simulink library "cdsDacKill"  (Simulink 7.5)
settings: Solver=ode45  StartTime=0.0  StopTime=10.0  RelTol=1e-3
settings Model: Creator=rolf.bork  LastModifiedBy=rolf.bork

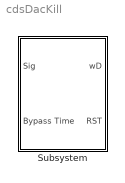
== system cdsDacKill ==
  Subsystem : Subsystem

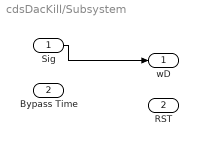
== system cdsDacKill/Subsystem ==
  Sig : Inport  OutDataType=fixdt(1, 16)  OutScaling=2^0
  Bypass Time : Inport  Port=2  OutDataType=fixdt(1, 16)  OutScaling=2^0
  wD : Outport  OutDataType=fixdt(1, 16)  OutScaling=2^0
  RST : Outport  Port=2  OutDataType=fixdt(1, 16)  OutScaling=2^0
  wires:
  Sig/1 -> wD/1
